simulink model "predball"  (Simulink 6.3)
settings: Solver=ode5  SolverMode=SingleTasking  StartTime=0.0  StopTime=30  FixedStep=0.01  RelTol=1e-3  AbsTol=1e-6
undefined symbols (not defined in the file or in its folder): now, sfunxy2
libraries: simulink3 x3
settings Model: Creator=eyarrow  LastModifiedBy=mbharadw  ExtModeTrigMode=oneshot  ExtModeArmWhenConnect=off  TunableVars=prueba  TunableVarsStorageClass=Auto  StrictBusMsg=None
settings DataIOCC: LimitDataPoints=off  SaveOutput=off  SignalLoggingName=sigsOut
settings OptimizationCC: BooleanDataType=off
settings DebuggingCC: SolverPrmCheckMsg=none
settings HardwareCC: TargetUnknown=on
settings RTWCC: TemplateMakefile=grt_vc.tmf

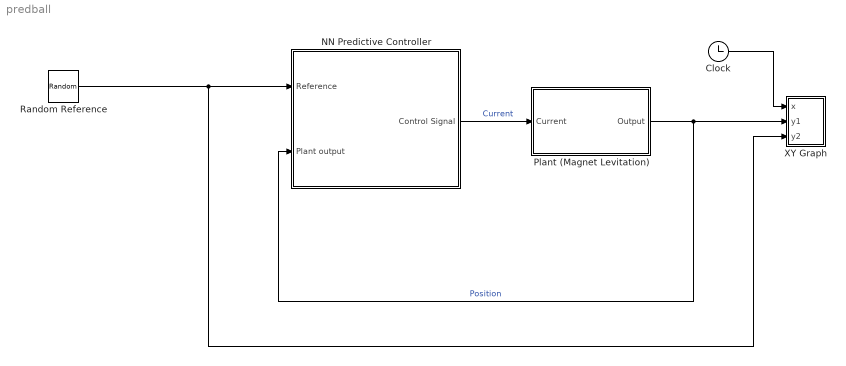
== system predball ==
  Clock : Clock
      settings: Decimation=10
  NN Predictive Controller : Subsystem  mask(NN Predictive Controller){N2=9, Nu=2, Ts=0.01, rho=0.005, alpha=0.001, csrchfun=csrchcha, maxiter=2, S1=9, Ni=3, Nj=2, sim_file=ballrepel0, trainfun=trainlm, Use_validation=1, Use_Testing=0, max_i=4, min_i=0, sam_training=10000, epochs=200, minp=0.013569924065719701, maxp=3.9919475548539087, mint=0.5, maxt=4.8553071923405362, Normalize=0, IW=[6.0992684989626964 -3.4057613377021299 2.8284879191363013;0.0031446091662587555 -0.0023677675323538839 -0.00062304892754021766;0.099266319350885812 0.048519647269651175 0.0025055386954869144;-0.0013445676464647707 0.00036889386984801059 -0.0030159166450831622;-1.0434582922964253 0.79109864730204449 0.91872153700183812;-0.00015255877173089871 0.00027144459111970941 0.0046690325671030018;0.4112390191083391 -0.99610766853970367 0.10432388168712149;-0.0094043572120226532 0.009710698502654342 -0.011307214003015112;-0.00032389016715114803 2.9262252362741224e-005 -0.0011856877339459133], LW1_2=[-0.75504663599627042 -0.40548770125984618;-0.91833066581615452 0.44462380813577707;-0.49150839323020501 0.25765411048438924;-0.11269530512343538 -0.18150834735330829;-0.33415698287239015 1.9376241402885785;-0.056845296032828375 0.38719752449976191;2.7052303570785732 -0.10850668752945752;-0.18472905081024196 -0.56254313245107257;0.36745424539455768 -0.27151820645760749], LW2_1=[-3.8454064803760212e-005 -1.0968850223149691 0.042826646017039456 -1.3151930617096832 -0.0002772064774394286 0.90141889537625086 -0.00276713044738676 -0.20145780532088417 5.313108837236447], B1=[2.1551700251490771;3.8509781495954791;-1.1007432449457728;1.4756440925383119;-2.9390167747519924;-0.41202014072175058;-0.47348766006921089;-0.12792175043576609;-0.068227544760648864], B2=3.0056846398281221, max_i_int=0.3, min_i_int=0.01, limit_output=1, max_output=Inf, min_output=0, Use_Previous_Weights=1}
      mask prompts: Ts "Sample time"; rho "rho (typically = 0.03)"; alpha "alpha (typically = 0.001)"; csrchfun "Minimization rutine"; trainfun "Training function"
      mask help: NN Predictive Controller. You first train a neural network model of the plant to be controlled. The controller uses the plant model to predict plant performance over a specified time horizon. An optimization algorithm determines the control signal that optimizes plant performance over this horizon. Double click the NN Predictive Controller block to train the plant model and set the controller parameters.
      mask init:
      | xl = [0   .53   .53     .85   .85  .53  .53  NaN .85  .92 .92];
      | yl = [.95 .95 1.05  1.05   .82  .82  .95  NaN  .95 .95 .65];
      | x2 = [0 .53    NaN .92 1.2 NaN .53 .85 .85 .53 .53 ];
      | y2 = [.39 .39   NaN .65 .65 NaN .59 .59 .29 .29  .59];
      | x3 = [.67 .67 NaN .64 .67 .70 NaN .53 .4   .4   .53 NaN .46 .53 .46];
      | y3 = [.59 .82 NaN .66 .59 .66 NaN .55 .55 .86 .86 NaN  .89 .86 .83];
      | 
      | x1t=.03; y1t=.31;
      | x2t=.03; y2t=.8;
      | x8t=.03;y8t=.21;
      | x3t=.77; y3t=.53;
      | x4t=.77; y4t=.44;
      | x5t=.45; y5t=.76;
      | x6t=.45; y6t=.35;
      | x7t=.45; y7t=.25;
      settings: OpenFcn=nncontrolutil('nnpredict','',gcbh,gcb);
      mask StyleString: edit,edit,edit,edit,edit,popup(csrchgol|csrchbac|csrchhyb|csrchbre|csrchcha),edit,edit,edit,edit,edit,popup(trainbfg|trainbr |traincgb|traincgf|traincgp|traingd|traingdm|traingda|traingdx|trainlm |trainoss|trainrp |trainscg),edit,edit,edit,edit,edit,edit,edit,edit,edit,edit,edit,edit,edit,edit,edit,edit,edit,edit,edit,edit,edit,edit
      mask Display:
      | plot([[xl NaN x2]*.9-.075 ], [[yl  NaN y2]*.9-.1 ]);
      | plot([[x3]*.9-.075 ], [[y3]*.9-.1 ]);
      | text(x1t,y1t,'Plant');
      | text(x8t,y8t,'Output');
      | text(x2t,y2t,'Reference');
      | text(x3t,y3t,'Control');
      | text(x4t,y4t,'Signal');
      | text(x5t,y5t,'Optim.');
      | text(x6t,y6t,'NN');
      | text(x7t,y7t,'Model');
  Plant (Magnet Levitation) : Subsystem
      mask init:
      | x1=[-2 -2 2 2 -2 NaN -2 -2 2 2 -2];
      | y1=[5 4 4 5 5 NaN 2 0 0 2 2];
      | x2=[-2 -2 2 2 -2 NaN -2   2  NaN -2 2 NaN 2    4    NaN 2  4];
      | y2=[4  3  3 4  4 NaN 1.5 1  NaN 1 .5 NaN 1.5 1.5 NaN .5 .5];
      | x1t = -.5 ; y1t = 4.4;
      | x2t = -.5; y2t = 3.4;
      mask Display:
      | plot([-10],[0],[10],[5]);
      | plot([x1 NaN x2],[y1 NaN y2]);
      | text(x1t,y1t,'N')
      | text(x2t,y2t,'S')
  Random Reference : UniformRandomNumber  Minimum=0.5  Maximum=3  Seed=round(now)  SampleTime=5
  XY Graph : Subsystem  LoadFcn=sfunxy2([],[],[],'LoadBlock')  StartFcn=sfunxy2([],[],[],'Start')  StopFcn=sfunxy2([],[],[],'Stop')  mask(XY scope.){xmin=0, xmax=5, ymin=0, ymax=2, st=-1}
      mask prompts: xmin "x-min:"; xmax "x-max:"; ymin "y-min:"; ymax "y-max:"; st "Sample time:"
      mask help: XY scope using MATLAB graph window. First input is used as time base. Enter plotting ranges.
      settings: CopyFcn=sfunxy2([],[],[],'CopyBlock')  DeleteFcn=sfunxy2([],[],[],'DeleteBlock')  NameChangeFcn=sfunxy2([],[],[],'NameChange')
      mask Help: This block can be used to explore limit cycles. Look at the function sfunxy.m to see how it works.
      mask Display: plot([.05 .95 .95 .05 .05],[.45 .45 .95 .95 .45], 0.5+cos(0:0.1:2*pi)*0.3,0.7+sin(0:0.1:2*pi)*0.2)
  wires:
  Random Reference/1 -> XY Graph/3(y2), NN Predictive Controller/1(Reference)
  Plant (Magnet Levitation)/1(Output) -> XY Graph/2(y1), NN Predictive Controller/2(Plant output)  "Position"
  Clock/1 -> XY Graph/1(x)
  NN Predictive Controller/1(Control Signal) -> Plant (Magnet Levitation)/1(Current)  "Current"

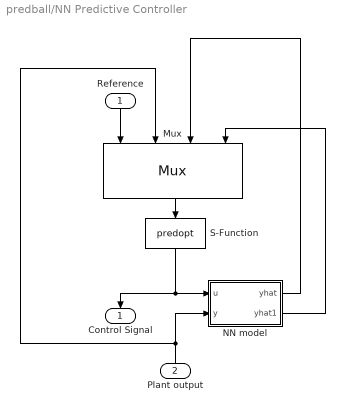
== system predball/NN Predictive Controller ==
  Reference : Inport  Orientation=down
  Plant output : Inport  Orientation=up  Port=2
  Mux : Mux  Orientation=down
      settings: DisplayOption=signals
  NN model : Subsystem
  S-Function : S-Function  Orientation=down  FunctionName=predopt  Parameters=N2,Ts,Nu,maxiter,csrchfun,rho,alpha,S1,IW,LW1_2,LW2_1,B1,B2,Ni,Nj,min_i,max_i,minp,maxp,mint,maxt,Normalize
  Control Signal : Outport  Orientation=down
  wires:
  Plant output/1 -> Mux/2, NN model/2(y)
  Reference/1 -> Mux/1
  NN model/1(yhat) -> Mux/3
  NN model/2(yhat1) -> Mux/4
  S-Function/1 -> Control Signal/1, NN model/1(u)
  Mux/1 -> S-Function/1

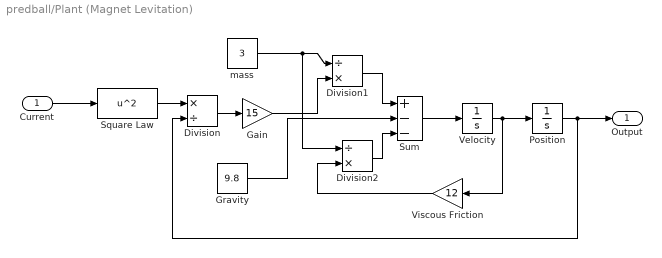
== system predball/Plant (Magnet Levitation) ==
  Current : Inport
  Division : Product  Inputs=*/  SaturateOnIntegerOverflow=on  InputSameDT=on
  Division1 : Product  Inputs=/*  SaturateOnIntegerOverflow=on  InputSameDT=on
  Division2 : Product  Inputs=/*  SaturateOnIntegerOverflow=on  InputSameDT=on
  Gain : Gain  Gain=15  SaturateOnIntegerOverflow=on
  Gravity : Constant  Value=9.8
  Position : Integrator  InitialCondition=.5
  Square Law : Fcn  Expr=u^2
  Sum : Sum  Inputs=|+--  SaturateOnIntegerOverflow=on  InputSameDT=on
  Velocity : Integrator
  Viscous Friction : Gain  Orientation=left  Gain=12  SaturateOnIntegerOverflow=on
  mass : Constant  Value=3
  Output : Outport
  wires:
  Position/1 -> Output/1, Division/2
  Current/1 -> Square Law/1
  Division2/1 -> Sum/3
  Viscous Friction/1 -> Division2/2
  mass/1 -> Division2/1, Division1/1
  Division1/1 -> Sum/1
  Gain/1 -> Division1/2
  Sum/1 -> Velocity/1
  Velocity/1 -> Viscous Friction/1, Position/1
  Gravity/1 -> Sum/2
  Division/1 -> Gain/1
  Square Law/1 -> Division/1

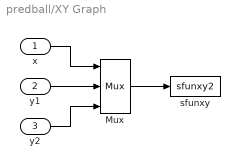
== system predball/XY Graph ==
  x : Inport
  y1 : Inport  Port=2
  y2 : Inport  Port=3
  Mux : Mux  Inputs=3
  sfunxy : S-Function  FunctionName=sfunxy2  Parameters=[xmin xmax ymin ymax], st
  wires:
  Mux/1 -> sfunxy/1
  x/1 -> Mux/1
  y1/1 -> Mux/2
  y2/1 -> Mux/3

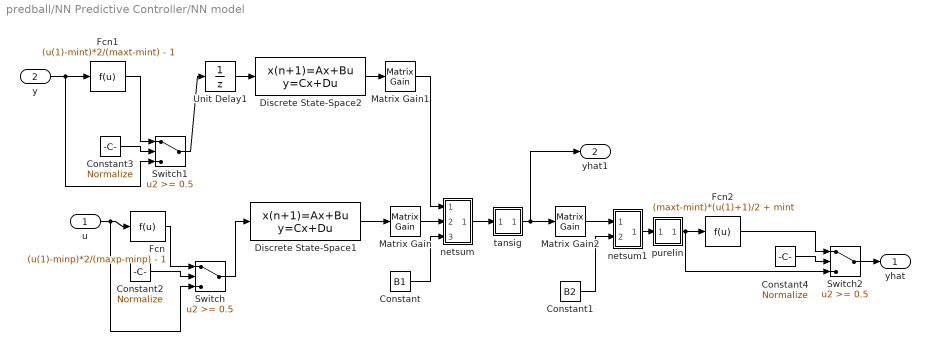
== system predball/NN Predictive Controller/NN model ==
  u : Inport
  y : Inport  Port=2
  Constant : Constant  Value=B1
  Constant1 : Constant  Value=B2
  Constant2 : Constant  Value=Normalize
  Constant3 : Constant  Value=Normalize
  Constant4 : Constant  Value=Normalize
  Discrete State-Space1 : DiscreteStateSpace  A=[zeros(1,Ni-1);eye(Ni-2,Ni-1)] %0 %[0 0;1 0]  B=eye(Ni-1,1) %1 %[1;0]  C=[zeros(1,Ni-1);eye(Ni-1,Ni-1)] %[0;1] %[1 0;0 1]  D="eye(Ni,1)  %[1;0] %[0;0]"  SampleTime=Ts
  Discrete State-Space2 : DiscreteStateSpace  A=[zeros(1,Nj-1);eye(Nj-2,Nj-1)] %0 %[0 0;1 0]  B=eye(Nj-1,1) %1 %[1;0]  C=[zeros(1,Nj-1);eye(Nj-1,Nj-1)] %[0;1] %[1 0;0 1]  D="eye(Nj,1)  %[1;0] %[0;0]"  SampleTime=Ts
  Fcn : Fcn  Expr=(u(1)-minp)*2/(maxp-minp) - 1
  Fcn1 : Fcn  Expr=(u(1)-mint)*2/(maxt-mint) - 1
  Fcn2 : Fcn  Expr=(maxt-mint)*(u(1)+1)/2 + mint
  Matrix Gain : simulink3/Math/Matrix Gain  K=IW
  Matrix Gain1 : simulink3/Math/Matrix Gain  K=LW1_2
  Matrix Gain2 : simulink3/Math/Matrix Gain  K=LW2_1
  Switch : Switch  Threshold=0.5  SaturateOnIntegerOverflow=on  InputSameDT=on
  Switch1 : Switch  Threshold=0.5  SaturateOnIntegerOverflow=on  InputSameDT=on
  Switch2 : Switch  Threshold=0.5  SaturateOnIntegerOverflow=on  InputSameDT=on
  Unit Delay1 : UnitDelay  SampleTime=Ts
  netsum : Subsystem
      mask Display: disp('+')
  netsum1 : Subsystem
      mask Display: disp('+')
  purelin : Subsystem
      mask Display: plot([-1 1],[0 0],[-1 1],[-1 1])
  tansig : Subsystem
      mask Display: plot([-1 1],[0 0],[-1 -.9 -.8 -.7 -.6 -.5 -.4 -.3 -.2 -.1 0 .1 .2 .3 .4 .5 .6 .7 .8 .9 1],2./(1+exp(-8*[-1 -.9 -.8 -.7 -.6 -.5 -.4 -.3 -.2 -.1 0 .1 .2 .3 .4 .5 .6 .7 .8 .9 1]))-1)
  yhat : Outport
  yhat1 : Outport  Port=2
  wires:
  purelin/1(a) -> Switch2/3, Fcn2/1
  Fcn2/1 -> Switch2/1
  Switch2/1 -> yhat/1
  Constant4/1 -> Switch2/2
  y/1 -> Switch1/3, Fcn1/1
  Fcn1/1 -> Switch1/1
  Switch1/1 -> Unit Delay1/1
  Constant3/1 -> Switch1/2
  Unit Delay1/1 -> Discrete State-Space2/1
  Discrete State-Space2/1 -> Matrix Gain1/1
  Constant2/1 -> Switch/2
  u/1 -> Switch/3, Fcn/1
  Switch/1 -> Discrete State-Space1/1
  Fcn/1 -> Switch/1
  Discrete State-Space1/1 -> Matrix Gain/1
  tansig/1(a) -> yhat1/1, Matrix Gain2/1
  Matrix Gain/1 -> netsum/2(In2)
  Matrix Gain1/1 -> netsum/1(In1)
  Constant/1 -> netsum/3(In3)
  netsum/1(Out1) -> tansig/1(n)
  Matrix Gain2/1 -> netsum1/1(In1)
  Constant1/1 -> netsum1/2(In2)
  netsum1/1(Out1) -> purelin/1(n)

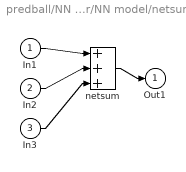
== system predball/NN Predictive Controller/NN model/netsum ==
  In1 : Inport
  In2 : Inport  Port=2
  In3 : Inport  Port=3
  netsum : Sum  Inputs=3  SaturateOnIntegerOverflow=on  InputSameDT=on
  Out1 : Outport
  wires:
  netsum/1 -> Out1/1
  In3/1 -> netsum/3
  In2/1 -> netsum/2
  In1/1 -> netsum/1

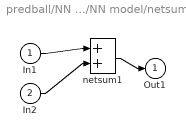
== system predball/NN Predictive Controller/NN model/netsum1 ==
  In1 : Inport
  In2 : Inport  Port=2
  netsum1 : Sum  Inputs=2  SaturateOnIntegerOverflow=on  InputSameDT=on
  Out1 : Outport
  wires:
  netsum1/1 -> Out1/1
  In2/1 -> netsum1/2
  In1/1 -> netsum1/1

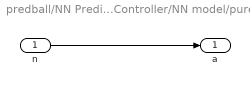
== system predball/NN Predictive Controller/NN model/purelin ==
  n : Inport
  a : Outport
  wires:
  n/1 -> a/1

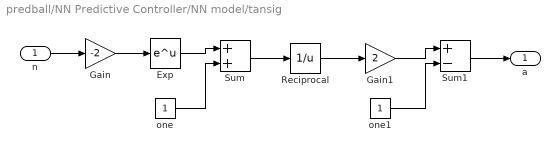
== system predball/NN Predictive Controller/NN model/tansig ==
  n : Inport
  Exp : Math  SaturateOnIntegerOverflow=on
  Gain : Gain  Gain=-2  SaturateOnIntegerOverflow=on
  Gain1 : Gain  Gain=2  SaturateOnIntegerOverflow=on
  Reciprocal : Math  Operator=reciprocal  SaturateOnIntegerOverflow=on
  Sum : Sum  SaturateOnIntegerOverflow=on  InputSameDT=on
  Sum1 : Sum  Inputs=+-  SaturateOnIntegerOverflow=on  InputSameDT=on
  one : Constant
  one1 : Constant
  a : Outport
  wires:
  Sum1/1 -> a/1
  one1/1 -> Sum1/2
  Gain1/1 -> Sum1/1
  Reciprocal/1 -> Gain1/1
  Sum/1 -> Reciprocal/1
  one/1 -> Sum/2
  Exp/1 -> Sum/1
  Gain/1 -> Exp/1
  n/1 -> Gain/1
